simulink model "ejercicio7_"  (R2012a)
settings: Solver=ode45  SolverMode=SingleTasking  StartTime=0.0  StopTime=10.0  RelTol=1e-3
values from neighbouring files (symbols this model uses):
  B = [0 0 ... (first row only)    [Problem_5_Matlab.m]    (also in anexo_parcial.m = [1/L 0 0 0 0]'; ejemplo_electrico.m = [1/L; 0]; ejemplo_mecanico.m = [0; 1/M1;0 ;0]; ejercicio7_taller2SM.m = [0 1/(M+J/R^2)]')
  J = 12    [ejercicio7_taller2SM.m]    (also in motord_DC_rot.m = 0.01)
  K1 = 700    [Problem_5_Matlab.m]    (also in ejemplo_mecanico.m = 100; ejercicio7_taller2SM.m = 34; grupo_roberto.m = 3; veengranes.m = 5)
  K2 = 20    [Problem_5_Matlab.m]    (also in ejercicio7_taller2SM.m = 300; grupo_roberto.m = 3; veengranes.m = 4)
  M = 20    [Problem_5_Matlab.m]    (also in ejercicio7_taller2SM.m = 10; grupo_roberto.m = 1)
  R = 10    [anexo_parcial.m]    (also in ejemplo_electrico.m = 1000; ejercicio7_taller2SM.m = 0.01; motord_DC_rot.m; nivel_tanque.m = 37)
settings Model: CovMetricSettings=dwe  CovHtmlReporting=off  covSaveCumulativeToWorkspaceVar=off  CovSaveSingleToWorkspaceVar=off  CovExternalEMLEnable=on  Creator=carma  LastModifiedBy=carma
settings DataIOCC: SaveFormat=StructureWithTime  ReturnWorkspaceOutputs=off
settings OptimizationCC: LifeSpan=inf  SimCompilerOptimization=Off
settings DebuggingCC: FcnCallInpInsideContextMsg=Enable All
settings HardwareCC: ProdWordSize=32  ProdHWDeviceType=Specified
settings SFSimCC: SimUseLocalCustomCode=off
settings RTWCC: RTWUseLocalCustomCode=off  RTWCompilerOptimization=Off
settings GRTTargetCC: CodeReplacementLibrary=C99 (ISO)  CPPClassGenCompliant=off

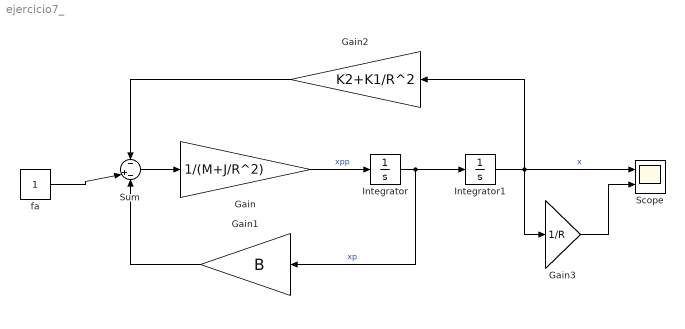
== system ejercicio7_ ==
  Gain : Gain  Gain=1/(M+J/R^2)
  Gain1 : Gain  Gain=B
  Gain2 : Gain  Gain=K2+K1/R^2
  Gain3 : Gain  Gain=1/R
  Integrator : Integrator
  Integrator1 : Integrator
  Scope : Scope  NumInputPorts=2
      settings: TimeRange=auto  MaxDataPoints=5000  SaveToWorkspace=off  SaveName=ScopeData  YMin=-10~-5  YMax=10~5  SampleTime=-1
  Sum : Sum  Inputs=-|+-
  fa : Constant
  wires:
  fa/1 -> Sum/2
  Sum/1 -> Gain/1
  Gain/1 -> Integrator/1  "xpp"
  Integrator/1 -> Gain1/1, Integrator1/1  "xp"
  Integrator1/1 -> Gain3/1, Gain2/1, Scope/1  "x"
  Gain1/1 -> Sum/3
  Gain2/1 -> Sum/1
  Gain3/1 -> Scope/2
